simulink model "untitled239"  (Simulink 8.9)
settings: Solver=VariableStepAuto  StartTime=0.0  StopTime=0.5  MaxStep=1e-4  RelTol=1e-3
libraries: powerlib x35
settings Model: Creator=laptop solutions lab  LastModifiedBy=laptop solutions lab
settings DataIOCC: LimitDataPoints=off  SaveFormat=Dataset  SignalLoggingSaveFormat=Dataset
settings OptimizationCC: LifeSpan=auto
settings DebuggingCC: UnderspecifiedInitializationDetection=Simplified  MergeDetectMultiDrivingBlocksExec=error  FcnCallInpInsideContextMsg=error  StateNameClashWarn=none  SFUnexpectedBacktrackingDiag=error  SFNoUnconditionalDefaultTransitionDiag=error  SFExecutionAtInitializationDiag=warning
settings HardwareCC: ProdBitPerPointer=64  ProdBitPerSizeT=64  ProdBitPerPtrDiffT=64  ProdLargestAtomicFloat=Float  ProdIntDivRoundTo=Zero  ProdEndianess=LittleEndian  ProdWordSize=64  ProdHWDeviceType=Intel->x86-64 (Windows64)
settings ModelReferenceCC: PropagateSignalLabelsOutOfModel=on
settings GRTTargetCC: TargetLangStandard=C99 (ISO)  GeneratePreprocessorConditionals=Use local settings  CombineOutputUpdateFcns=on  GRTInterface=off
settings ConfigComp: CovMetricSettings=dwe  CovHtmlReporting=off  CovSaveCumulativeToWorkspaceVar=off  CovSaveSingleToWorkspaceVar=off  CovExternalEMLEnable=on

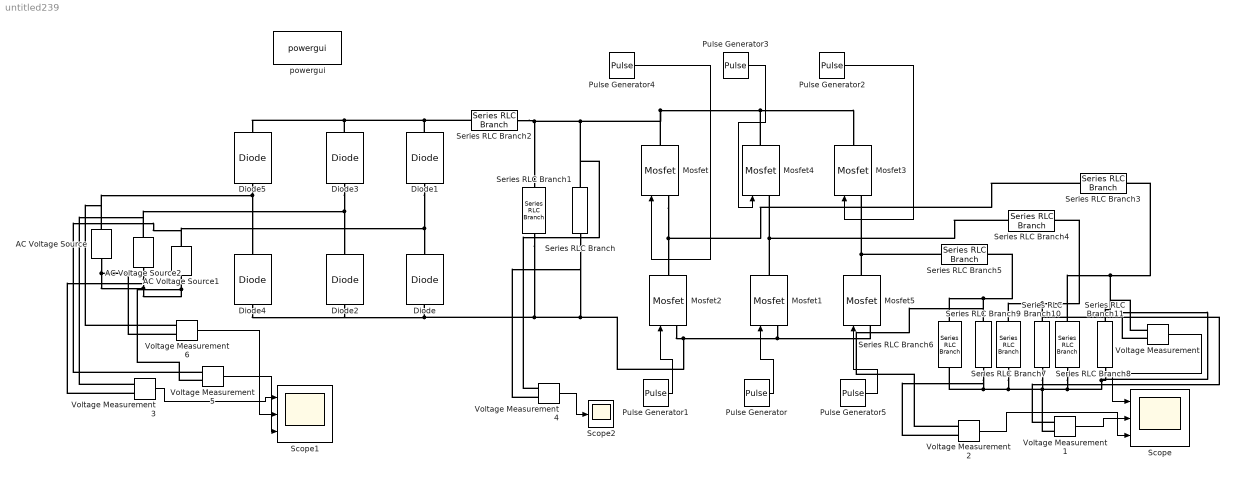
== system untitled239 ==
  AC Voltage Source : powerlib/Electrical Sources/AC Voltage Source  Amplitude=100  Phase=0  Frequency=50  SampleTime=0  Measurements=None  BusType=swing  Pref=10e3  Qref=0  Qmin=-inf  Qmax=+inf
  AC Voltage Source1 : powerlib/Electrical Sources/AC Voltage Source  Amplitude=100  Phase=240  Frequency=50  SampleTime=0  Measurements=None  BusType=swing  Pref=10e3  Qref=0  Qmin=-inf  Qmax=+inf
  AC Voltage Source2 : powerlib/Electrical Sources/AC Voltage Source  Amplitude=100  Phase=120  Frequency=50  SampleTime=0  Measurements=None  BusType=swing  Pref=10e3  Qref=0  Qmin=-inf  Qmax=+inf
  Diode{,1..5} (6 alike) : powerlib/Power Electronics/Diode  Ron=0.001  Lon=0  Vf=0.8  IC=0  UseSnubber=0  Rs=500  Cs=250e-9  Measurements=off
  Mosfet{,1..5} (6 alike) : powerlib/Power Electronics/Mosfet  Ron=0.1  Lon=0  Rd=0.01  Vfd=0  IC=0  Rs=1e5  Cs=inf  Measurements=off
  Pulse Generator : DiscretePulseGenerator  PulseType=Time based  Period=1/130  PulseWidth=50  PhaseDelay=300/(130*360)
  Pulse Generator1 : DiscretePulseGenerator  PulseType=Time based  TimeSource=Use external signal  Period=1/130  PulseWidth=50  PhaseDelay=180/(130*360)
  Pulse Generator2 : DiscretePulseGenerator  PulseType=Time based  Period=1/130  PulseWidth=50  PhaseDelay=240/(130*360)
  Pulse Generator3 : DiscretePulseGenerator  PulseType=Time based  Period=1/130  PulseWidth=50  PhaseDelay=120/(130*360)
  Pulse Generator4 : DiscretePulseGenerator  PulseType=Time based  Period=1/130  PulseWidth=50
  Pulse Generator5 : DiscretePulseGenerator  PulseType=Time based  Period=1/130  PulseWidth=50  PhaseDelay=60/(130*360)
  Scope : Scope  NumInputPorts=3
  Scope1 : Scope  NumInputPorts=3
  Scope2 : Scope
  Series RLC Branch{,9..11} (4 alike) : powerlib/Elements/Series RLC Branch  LConnTagsString=__new0  RConnTagsString=__new0  BranchType=R  Resistance=50  Inductance=1e-3  SetiL0=off  InitialCurrent=0  Capacitance=1e-6  Setx0=off  InitialVoltage=0  Measurements=None
  Series RLC Branch1 : powerlib/Elements/Series RLC Branch  LConnTagsString=__new0  RConnTagsString=__new0  BranchType=C  Resistance=1  Inductance=1e-3  SetiL0=off  InitialCurrent=0  Capacitance=0.01013  Setx0=off  InitialVoltage=0  Measurements=None
  Series RLC Branch{2..5} (4 alike) : powerlib/Elements/Series RLC Branch  LConnTagsString=__new0  RConnTagsString=__new0  BranchType=L  Resistance=1  Inductance=1e-3  SetiL0=off  InitialCurrent=0  Capacitance=1e-6  Setx0=off  InitialVoltage=0  Measurements=None
  Series RLC Branch6 : powerlib/Elements/Series RLC Branch  LConnTagsString=__new0  RConnTagsString=__new0  BranchType=C  Resistance=1  Inductance=1e-3  SetiL0=off  InitialCurrent=0  Capacitance=1.49e-3  Setx0=off  InitialVoltage=0  Measurements=None
  Series RLC Branch7 : powerlib/Elements/Series RLC Branch  LConnTagsString=__new0  RConnTagsString=__new0  BranchType=C  Resistance=1  Inductance=1e-3  SetiL0=off  InitialCurrent=0  Capacitance=1.49e-3  Setx0=off  InitialVoltage=0  Measurements=None
  Series RLC Branch8 : powerlib/Elements/Series RLC Branch  LConnTagsString=__new0  RConnTagsString=__new0  BranchType=C  Resistance=1  Inductance=1e-3  SetiL0=off  InitialCurrent=0  Capacitance=1.49e-3  Setx0=off  InitialVoltage=0  Measurements=None
  Voltage Measurement{,1..6} (7 alike) : powerlib/Measurements/Voltage Measurement  PhasorSimulation=off  OutputType=Complex  PSBequivalent=0
  powergui : powerlib/powergui  Priority=1  SimulationMode=Continuous  SampleTime=50e-6  frequency=60  Iterations=50  frequencyindice=50  Pbase=100e6  ErrMax=1e-4  UnitsV=kV  UnitsW=MW  buscounter=0  FunctionMessages=off  echomessages=off  EnableUseOfTLC=off  CurrentSourceSwitches=off  DisableSnubberDevices=off  DisableRonSwitches=off  DisableVfSwitches=off  DisplayEquations=off  SolverType=Tustin/Backward Euler (TBE)  Interpol=off  ExternalGateDelay=off  methode=off  Ts=100  x0status=blocks  SPID=on  SwTol=0  HookPort=off  RestoreLinks=warning  ResistiveCurrentMeasurement=off  Frange=[0:2:500]  Ylog=off  Xlog=on  ShowGrid=off  save=off  variable=ZData  structure=0  ZoomFFT=off  StartTime=0.0  cycles=1  DisplayStyle=1  fundamental=60  FreqAxis=off  MaxFrequency=1000  frequencyindicesteady=1  RmsSteady=1  display=off
  wires:
  Pulse Generator4/1 -> Mosfet/1
  Pulse Generator3/1 -> Mosfet4/1
  Pulse Generator2/1 -> Mosfet3/1
  Pulse Generator1/1 -> Mosfet2/1
  Pulse Generator/1 -> Mosfet1/1
  Pulse Generator5/1 -> Mosfet5/1
  Voltage Measurement/1 -> Scope/1
  Voltage Measurement1/1 -> Scope/2
  Voltage Measurement2/1 -> Scope/3
  Voltage Measurement4/1 -> Scope2/1
  Voltage Measurement3/1 -> Scope1/1
  Voltage Measurement6/1 -> Scope1/2
  Voltage Measurement5/1 -> Scope1/3
  connections:
  Diode5/LConn1 -- Voltage Measurement6/LConn1 -- AC Voltage Source/RConn1 -- Diode4/RConn1
  Diode3/LConn1 -- Voltage Measurement3/LConn1 -- AC Voltage Source2/RConn1 -- Diode2/RConn1
  Diode1/LConn1 -- Voltage Measurement5/LConn1 -- AC Voltage Source1/RConn1 -- Diode/RConn1
  Diode1/RConn1 -- Diode3/RConn1 -- Diode5/RConn1 -- Series RLC Branch2/LConn1
  Mosfet2/LConn1 -- Voltage Measurement4/LConn2 -- Series RLC Branch/RConn1 -- Diode2/LConn1 -- Diode4/LConn1 -- Diode/LConn1 -- Series RLC Branch1/RConn1 -- Mosfet1/LConn1 -- Mosfet5/LConn1
  Mosfet/RConn1 -- Voltage Measurement4/LConn1 -- Series RLC Branch/LConn1 -- Series RLC Branch1/LConn1 -- Series RLC Branch2/RConn1 -- Mosfet4/RConn1 -- Mosfet3/RConn1
  AC Voltage Source/LConn1 -- Voltage Measurement6/LConn2 -- Voltage Measurement3/LConn2 -- AC Voltage Source2/LConn1 -- Voltage Measurement5/LConn2 -- AC Voltage Source1/LConn1
  Mosfet/LConn1 -- Series RLC Branch3/LConn1 -- Mosfet2/RConn1
  Mosfet1/RConn1 -- Series RLC Branch4/LConn1 -- Mosfet4/LConn1
  Mosfet5/RConn1 -- Series RLC Branch5/LConn1 -- Mosfet3/LConn1
  Series RLC Branch11/RConn1 -- Voltage Measurement/LConn2 -- Series RLC Branch8/RConn1 -- Voltage Measurement1/LConn2 -- Series RLC Branch10/RConn1 -- Series RLC Branch7/RConn1 -- Voltage Measurement2/LConn2 -- Series RLC Branch9/RConn1 -- Series RLC Branch6/RConn1
  Series RLC Branch6/LConn1 -- Voltage Measurement2/LConn1 -- Series RLC Branch9/LConn1 -- Series RLC Branch5/RConn1
  Series RLC Branch7/LConn1 -- Voltage Measurement1/LConn1 -- Series RLC Branch10/LConn1 -- Series RLC Branch4/RConn1
  Series RLC Branch8/LConn1 -- Voltage Measurement/LConn1 -- Series RLC Branch11/LConn1 -- Series RLC Branch3/RConn1
